simulink model "nochange"  (R2022b)
settings: Solver=FixedStepDiscrete  StartTime=0.0  StopTime=10.0  FixedStep=1e-3  RelTol=1e-3
settings Model: Creator=ahmed  LastModifiedBy=ahmed

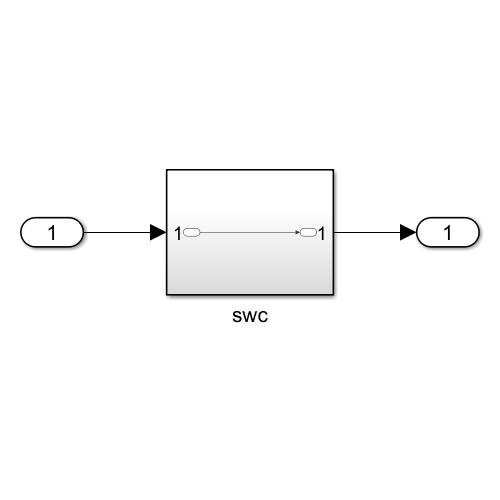
[thumbnail: Simulink's stored preview of the top-level diagram]
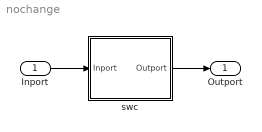
== system nochange ==
  Inport : Inport
  swc : Subsystem
  Outport : Outport
  wires:
  Inport/1 -> swc/1(Inport)
  swc/1(Outport) -> Outport/1

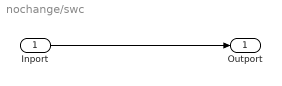
== system nochange/swc ==
  Inport : Inport
  Outport : Outport
  wires:
  Inport/1 -> Outport/1
